simulink model "cart_pendulum"  (R2020b)
settings: Solver=VariableStepAuto  StartTime=0.0  StopTime=10.0  RelTol=1e-3
values from neighbouring files (symbols this model uses):
  h = 0.01    [main_cart_pendulum_dlqr.m]
  maxforce = 50    [main_cart_pendulum_dlqr.m]
  setpoint = 0.5    [main_cart_pendulum_dlqr.m]
  x0 = [0; deg2rad(60); 0; 0]    [main_cart_pendulum_dlqr.m]
undefined symbols (not defined in the file or in its folder): add_states, lstates, ubar, xbar
libraries: cstblocks x1
settings Model: Creator=Kingdel  LastModifiedBy=Usuario

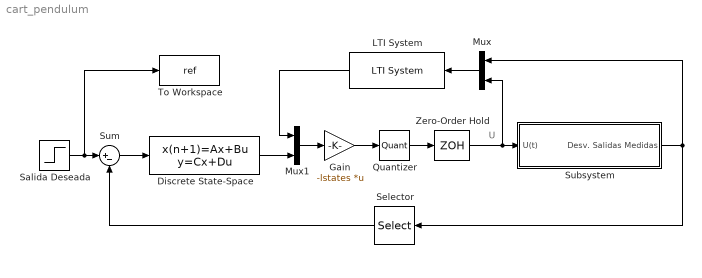
== system cart_pendulum ==
  note: U
  Discrete State-Space : DiscreteStateSpace  A=add_states.A  B=add_states.B  C=eye(size(add_states.A))  D=zeros(size(add_states.B))  SampleTime=h
  Gain : Gain  Gain=-lstates  Multiplication=Matrix(K*u) (u vector)
  LTI System : cstblocks/LTI System  sys=observer  IC=[]
  Mux : Mux  Inputs=2
  Mux1 : Mux  Inputs=2
  Quantizer : Quantizer  QuantizationInterval=qforce
  Salida Deseada : Step  Time=0  After=setpoint  SampleTime=h
  Selector : Selector  InputPortWidth=2  IndexOptions=Index vector (dialog)  Indices=1  OutputSizes=1
  Subsystem : Subsystem
  Sum : Sum  Inputs=|+-
  To Workspace : ToWorkspace  VariableName=ref  SaveFormat=Structure With Time  SampleTime=h
  Zero-Order Hold : ZeroOrderHold  SampleTime=h
  wires:
  Salida Deseada/1 -> To Workspace/1, Sum/1
  Zero-Order Hold/1 -> Mux/2, Subsystem/1(U(t))
  Mux1/1 -> Gain/1
  LTI System/1 -> Mux1/1
  Subsystem/1(Desv. Salidas Medidas) -> Mux/1, Selector/1
  Discrete State-Space/1 -> Mux1/2
  Sum/1 -> Discrete State-Space/1
  Selector/1 -> Sum/2
  Mux/1 -> LTI System/1
  Quantizer/1 -> Zero-Order Hold/1
  Gain/1 -> Quantizer/1

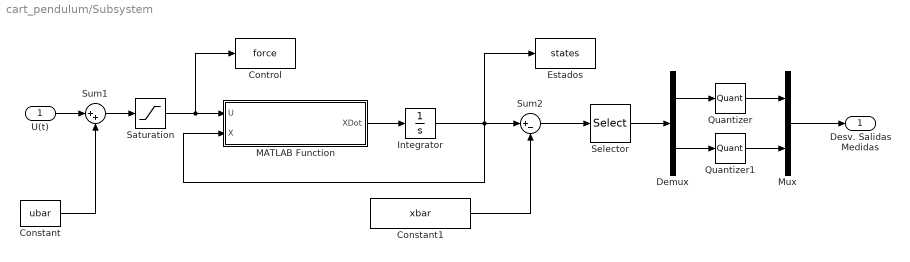
== system cart_pendulum/Subsystem ==
  U(t) : Inport
  Constant : Constant  Value=ubar
  Constant1 : Constant  Value=xbar
  Control : ToWorkspace  VariableName=force  SaveFormat=Structure With Time  SampleTime=h
  Demux : Demux  Outputs=2
  Estados : ToWorkspace  VariableName=states  SaveFormat=Structure With Time  SampleTime=h
  Integrator : Integrator  InitialCondition=x0
  MATLAB Function : MATLAB Function  TreatAsAtomicUnit=on
  Mux : Mux  Inputs=2
  Quantizer : Quantizer  QuantizationInterval=qposition
  Quantizer1 : Quantizer  QuantizationInterval=qangle
  Saturation : Saturate  UpperLimit=maxforce  LowerLimit=-maxforce
  Selector : Selector  InputPortWidth=4  IndexOptions=Index vector (dialog)  Indices=[1 2]  OutputSizes=1
  Sum1 : Sum  Inputs=|++
  Sum2 : Sum  Inputs=|+-
  Desv. Salidas Medidas : Outport  VectorParamsAs1DForOutWhenUnconnected=off
  wires:
  MATLAB Function/1(XDot) -> Integrator/1
  Integrator/1 -> MATLAB Function/2(X), Sum2/1, Estados/1
  Constant1/1 -> Sum2/2
  Constant/1 -> Sum1/2
  U(t)/1 -> Sum1/1
  Saturation/1 -> Control/1, MATLAB Function/1(U)
  Sum1/1 -> Saturation/1
  Selector/1 -> Demux/1
  Mux/1 -> Desv. Salidas Medidas/1
  Sum2/1 -> Selector/1
  Quantizer/1 -> Mux/1
  Demux/1 -> Quantizer/1
  Quantizer1/1 -> Mux/2
  Demux/2 -> Quantizer1/1

== matlab function cart_pendulum/Subsystem/MATLAB Function ==
  data: U input; XDot output; X input
function XDot = derivatives_of_states(U,X)
%#codegen
% Constants of the model
[M,m,J,L,a,g] = deal(1,0.1,0.025,0.5,0.5,9.807);
[X1,X2,X3,X4] = deal(X(1),X(2),X(3),X(4));

% Inertia matrix
D           = [M+m,-m*a*L*sin(X2);-m*a*L*sin(X2),m*a^2*L^2+J];

% Coriolis and centrifugal forces
H           = [-m*a*L*cos(X2)*X4^2; +m*a*L*g*cos(X2)];

% Impact detection
F           = impact_force(M+m,X1,X3);
U           = U + F;

% Generalized effort
E           = [U; 0];

% State space model
% x1 = x, x2 = theta, x3 = xdot, x4 = thetadot
XDot        = [X3; X4; D\(E-H)];
end

% Force for left impact
function F  = impact_force(Mass,Pos,Vel)
% Settling time
Ts          = 0.01;
% Damping 
Xi          = 0.707;
% Natural frequency
Wn          = 4/(Ts*Xi);
% Spring constant
Kp          = Mass*Wn^2;
% Damper constant
Kv          = 2*Mass*Xi*Wn;
F           = 0;
% Impact force
Limit       = 1.7;
if Pos < -Limit && Vel < 0
    F       = -Kp*(Pos+Limit) -Kv*Vel;
elseif Pos > Limit && Vel > 0
    F       = -Kp*(Pos-Limit) -Kv*Vel;
end
end
